simulink model "simple_blinking"  (R2017a)
settings: Solver=VariableStepAuto  StartTime=0.0  StopTime=10.0  RelTol=1e-3
settings Model: Creator=mini  LastModifiedBy=mini
settings OptimizationCC: BlockReduction=off  ConditionallyExecuteInputs=off  DefaultParameterBehavior=Inlined
settings DebuggingCC: AlgebraicLoopMsg=error
settings HardwareCC: ProdBitPerPointer=32  ProdBitPerSizeT=32  ProdBitPerPtrDiffT=32  ProdLargestAtomicFloat=None  ProdIntDivRoundTo=Undefined  ProdEndianess=Unspecified  ProdWordSize=32  ProdHWDeviceType=ASIC/FPGA->ASIC/FPGA  TargetBitPerPointer=64  TargetBitPerSizeT=64  TargetBitPerPtrDiffT=64  TargetLongLongMode=on  TargetIntDivRoundTo=Zero  TargetEndianess=LittleEndian  TargetWordSize=64  TargetHWDeviceType=MATLAB Host  ProdEqTarget=off

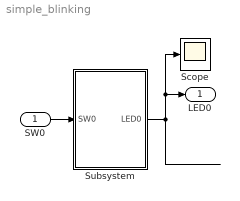
== system simple_blinking ==
  SW0 : Inport  OutDataTypeStr=boolean
  Scope : Scope
  Subsystem : Subsystem  TreatAsAtomicUnit=on
  LED0 : Outport  SampleTime=1
  wires:
  Subsystem/1(LED0) -> Scope/1, LED0/1
  SW0/1 -> Subsystem/1(SW0)

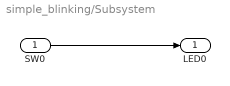
== system simple_blinking/Subsystem ==
  SW0 : Inport  OutDataTypeStr=boolean
  LED0 : Outport  SampleTime=1
  wires:
  SW0/1 -> LED0/1
